simulink model "gnc_ministack"  (R2025a)
settings: Solver=ode45  StartTime=0.0  StopTime=85  RelTol=1e-3
StartFcn:
  | startup()
libraries: sim3dlib x1, aerolibsim3d x1
settings Model: Creator=Jackt  LastModifiedBy=Jackt

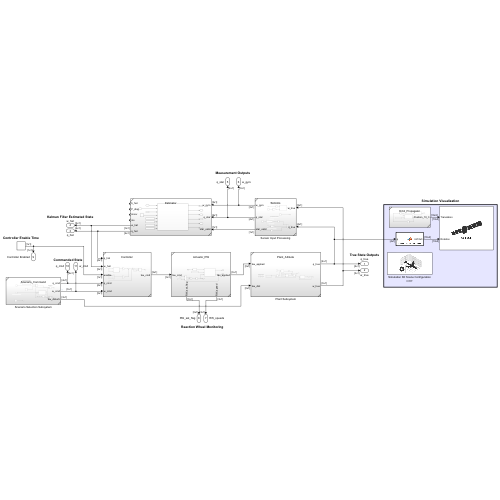
[thumbnail: Simulink's stored preview of the top-level diagram]
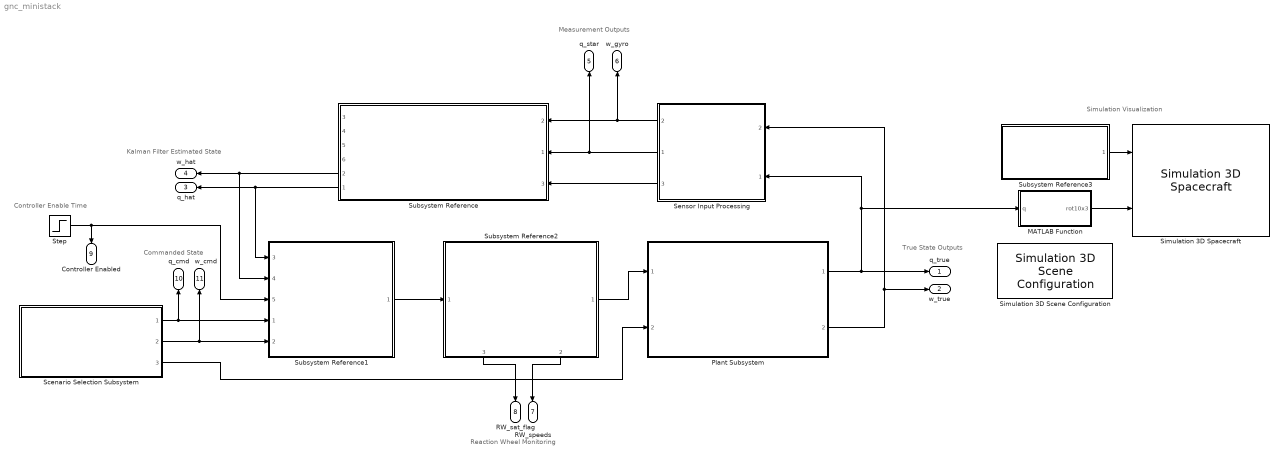
== system gnc_ministack ==
  note: Commanded State
  note: Controller Enable Time
  note: Reaction Wheel Monitoring
  note: Simulation Visualization
  note: Measurement Outputs
  note: True State Outputs
  note: Kalman Filter Estimated State
  MATLAB Function : MATLAB Function  TreatAsAtomicUnit=on
  Plant Subsystem : Subsystem  ReferencedSubsystem=Plant_Attitude
  Scenario Selection Subsystem : Subsystem  ReferencedSubsystem=Scenario_Command
  Sensor Input Processing : Subsystem  ReferencedSubsystem=Sensors
      settings: PortSchema="{\"entries\":[{\"content\":{\"sides\":[{\"content\":{\"connectorIds\":[\"In2\",\"In1\"]},\"type\":\"ConnectorPlacement.EquallySpacedRectSide\",\"uuid\":\"c1e9cccd-a19b-49d9-bc23-c04dc12a4bb5\"},{\"content\":{\"connectorIds\":[\"Out2\",\"Out1\",\"Out3\"],\"side\":\"RIGHT\"},\"type\":\"ConnectorPlacement.EquallySpacedRectSide\",\"uuid\":\"d99cdc6b-e9ef-4ed5-80da-dd2badbe997a\"},{\"content\":{\"side\":\"TOP\"},\"type\":\"ConnectorPlacement.EquallySpacedRectSide\",\"uuid\":\"ee231260-93e9-44f5-bf52-f5add3775a1d\"}]},\"type\":\"ConnectorPlacement.EquallySpacedConnector\",\"uuid\":\"7e127460-3e6f-4f82-b424-e04fed54d7b3\"}],\"packageUris\":[\"http://schema.mathworks.com/mf0/Connector/R2020b\"],\"version\":\"1.0\"}"
  Simulation 3D Scene Configuration : sim3dlib/Simulation 3D Scene Configuration  Priority=0  ProjectFormat=Default Scenes  SceneDesc=Earth  ProjectName=C:\Program Files\MATLAB\R2025a\toolbox\shared\sim3d_projects\automotive_project_windows\UE\WindowsNoEditor\VehicleSimulation.exe  ScenePath=/Game/Maps/HwStrght  EnableOpenDRIVE=off  vehTagList={'Custom';'Scene Origin';'SimulinkVehicle1'}  vehTag=SimulinkVehicle1  AttachedCameraRelativeTranslation=[0 0 0]  FreeCameraDefaultInitialTranslation=[-14000000, 0, 0]  AttachedCameraRelativeRotation=[0 0 0]  FreeCameraDefaultInitialRotation=[0, 0, 0]  ViewpointName=Custom  FreeCameraInitialTranslation=[-6, 0, 2]  ViewpointTranslation=[0 0 0]  FreeCameraInitialRotation=[0, -15, 0]  ViewpointRotation=[0 0 0]  OpVisEn=off  Ts=.02  EnableWindow=on  EnableRemoteAccess=off  EnableWeather=on  SunAzimuth=284.400  SunAltitude=40.0  EnableGeospatialSun=off  Latitude=0  Longitude=0  Date=2023-01-01  Time=10:30:00  GeoTimeZone=-5.0  SunDaylightSaving=off  wind=1  clouds=10  EnableVolumetricClouds=off  CloudCoverage=0  CloudAltitude=6  fog=0  rain=0  RaindropsEffect=off  SnowDensity=0  EnableGeospatial=off  TilesetSource=Earth terrain  UseTrueOrigin=off  OriginHeight=30000  OriginLatitude=40.744652  OriginLongitude=-73.988864  MapStyle=Aerial  AdditionalAssetIDs=[]  UseAdvancedSunSky=off  SolarTime=11  TimeZone=-5  Day=21  Month=9  Year=2022  UseDaylightSavingTime=off  DSTStartDay=10  DSTStartMonth=3  DSTEndDay=3  DSTEndMonth=11  DSTSwitchHour=2  sensorTag=MainCamera1  sensorId=1  sensorName=MainCamera1  mountLoc=Origin  offsetFlag=off  tmountOffset=[0, 0, 0]  rmountOffset=[0, 0, 0]  HorizontalResolution=1280  VerticalResolution=720  HorizontalFOV=60  mountPoint=[0 0 0]  mountOrientation=[0 0 0]  aMode=0  ID=1  GeoTrigger=Inactive  ViewNameList={'Custom'}  ViewTranslationList={'[-6 0 2]'}  ViewRotationList={'[0 -15 0]'}
      settings: AttributesFormatString=ICRF  LibrarySourceBlock=aerolibsim3d/Simulation 3D Scene Configuration
  Simulation 3D Spacecraft : aerolibsim3d/Simulation 3D Spacecraft  Priority=-1  Mesh=CubeSat  MeshPath=/MathWorksAerospaceContent/Vehicles/Spacecraft/CubeSat/Mesh/SK_CubeSat.SK_CubeSat  MeshPathSmall=/MathWorksAerospaceContent/Vehicles/Spacecraft/SmallSat/Mesh/SK_SmallSat.SK_SmallSat  SpacecraftColor=Silver  ActorName=SimulinkVehicle1  Translation=zeros(10, 3)  Rotation=zeros(10, 3)  ScaleInputPort=Dialog  Scale=[1 1 1]  InitialScale=[1 1 1]  IsGHSensorEnabled=off  AreGHRaysVisible=off  IsOutputReshapeEnabled=on  GHRayLength=1524  GHBodyOffset=1  GHContactLocation1=[0 0 0]  GHContactLocation2=[0 0 0]  GHContactLocation3=[0 0 0]  GHContactLocation4=[0 0 0]  WoWSensorTolerance=0.05  SampleTime=-1  ActorType=SimulinkVehicle  ID=1  aMode=0  ActorTag=SimulinkVehicle1
  Step : Step  Time=0  Before=1  SampleTime=0  VectorParams1D=off
  Subsystem Reference : Subsystem  ReferencedSubsystem=Estimator
      settings: PortSchema="{\"entries\":[{\"content\":{\"sides\":[{\"content\":{\"connectorIds\":[\"In2\",\"In1\",\"In3\"]},\"type\":\"ConnectorPlacement.EquallySpacedRectSide\",\"uuid\":\"6ff88212-69d9-4c32-a110-b4128dbcbd58\"},{\"content\":{\"connectorIds\":[\"Out3\",\"Out4\",\"Out5\",\"Out6\",\"Out2\",\"Out1\"],\"side\":\"RIGHT\"},\"type\":\"ConnectorPlacement.EquallySpacedRectSide\",\"uuid\":\"13b22769-b1cf-40a2-97ae-fd353d8761f4\"},{\"content\":{\"side\":\"TOP\"},\"type\":\"ConnectorPlacement.EquallySpacedRectSide\",\"uuid\":\"80c1570c-552a-494f-85a9-3ba650112d27\"}]},\"type\":\"ConnectorPlacement.EquallySpacedConnector\",\"uuid\":\"37c5906b-3676-4ab4-a32b-12b3e3b6617e\"}],\"packageUris\":[\"http://schema.mathworks.com/mf0/Connector/R2020b\"],\"version\":\"1.0\"}"
  Subsystem Reference1 : Subsystem  ReferencedSubsystem=Controller
      settings: PortSchema="{\"entries\":[{\"content\":{\"sides\":[{\"content\":{\"connectorIds\":[\"In3\",\"In4\",\"In5\",\"In1\",\"In2\"]},\"type\":\"ConnectorPlacement.EquallySpacedRectSide\",\"uuid\":\"50b51f02-92a3-4895-831f-474087d70428\"},{\"content\":{\"connectorIds\":[\"Out1\"],\"side\":\"RIGHT\"},\"type\":\"ConnectorPlacement.EquallySpacedRectSide\",\"uuid\":\"95d54d9e-6673-49b8-8b0a-15f9a2d5d6ed\"},{\"content\":{\"side\":\"TOP\"},\"type\":\"ConnectorPlacement.EquallySpacedRectSide\",\"uuid\":\"9b2dfc11-3477-4b71-bffc-31b65fad140d\"}]},\"type\":\"ConnectorPlacement.EquallySpacedConnector\",\"uuid\":\"333a9d20-5e34-4443-bcbe-37e2758feffc\"}],\"packageUris\":[\"http://schema.mathworks.com/mf0/Connector/R2020b\"],\"version\":\"1.0\"}"
  Subsystem Reference2 : Subsystem  ReferencedSubsystem=Actuator_RW
      settings: PortSchema="{\"entries\":[{\"content\":{\"sides\":[{\"content\":{\"connectorIds\":[\"In1\"]},\"type\":\"ConnectorPlacement.EquallySpacedRectSide\",\"uuid\":\"970f40e1-f7ca-420b-8ec9-a2b921625748\"},{\"content\":{\"connectorIds\":[\"Out1\"],\"side\":\"RIGHT\"},\"type\":\"ConnectorPlacement.EquallySpacedRectSide\",\"uuid\":\"35de2d62-f31e-438d-9acc-19246649a370\"},{\"content\":{\"side\":\"TOP\"},\"type\":\"ConnectorPlacement.EquallySpacedRectSide\",\"uuid\":\"82a92509-4f7d-481c-8e84-283404e2f7d8\"},{\"content\":{\"connectorIds\":[\"Out3\",\"Out2\"],\"side\":\"BOTTOM\"},\"type\":\"ConnectorPlacement.EquallySpacedRectSide\",\"uuid\":\"b07604dc-8104-479b-9fb4-03ecbc98cb9a\"}]},\"type\":\"ConnectorPlacement.EquallySpacedConnector\",\"uuid\":\"d401c8d7-6003-4b17-a86f-c889bdabed91\"}],\"packageUris\":[\"http://schema.mathworks.com/mf0/Connector/R2020b\"],\"version\":\"1.0\"}"
  Subsystem Reference3 : Subsystem  ReferencedSubsystem=Orbit_Propagator
  q_true : Outport
  w_true : Outport  Port=2
  q_hat : Outport  Port=3
  w_hat : Outport  Port=4
  q_star : Outport  Port=5
  w_gyro : Outport  Port=6
  RW_speeds : Outport  Port=7
  RW_sat_flag : Outport  Port=8
  Controller Enabled : Outport  Port=9
  q_cmd : Outport  Port=10
  w_cmd : Outport  Port=11
  wires:
  Plant Subsystem/1 -> Sensor Input Processing/1, MATLAB Function/1(q), q_true/1
  Plant Subsystem/2 -> w_true/1, Sensor Input Processing/2
  Scenario Selection Subsystem/1 -> Subsystem Reference1/1, q_cmd/1
  Scenario Selection Subsystem/2 -> w_cmd/1, Subsystem Reference1/2
  Subsystem Reference1/1 -> Subsystem Reference2/1
  Scenario Selection Subsystem/3 -> Plant Subsystem/2
  Sensor Input Processing/1 -> q_star/1, Subsystem Reference/1
  Sensor Input Processing/2 -> Subsystem Reference/2, w_gyro/1
  Sensor Input Processing/3 -> Subsystem Reference/3
  Subsystem Reference/1 -> Subsystem Reference1/3, q_hat/1
  Subsystem Reference/2 -> Subsystem Reference1/4, w_hat/1
  Subsystem Reference2/1 -> Plant Subsystem/1
  Subsystem Reference2/2 -> RW_speeds/1
  Subsystem Reference2/3 -> RW_sat_flag/1
  Step/1 -> Subsystem Reference1/5, Controller Enabled/1
  MATLAB Function/1(rot10x3) -> Simulation 3D Spacecraft/2
  Subsystem Reference3/1 -> Simulation 3D Spacecraft/1

== matlab function gnc_ministack/MATLAB Function ==
  data: q input; rot10x3 output
function rot10x3 = pack_cubesat_rpy(q)
% q: [4x1] scalar-first quaternion (assumed unit-ish)
% rot10x3: [10x3] rows are bones; row1 is BODY [roll pitch yaw] rad

q = q(:);
q = q / max(norm(q), 1e-12);

% Optional: stabilize sign to reduce visual "flips"
if q(1) < 0
    q = -q;
end

% Convert quaternion -> roll/pitch/yaw (ZYX yaw-pitch-roll)
q0=q(1); q1=q(2); q2=q(3); q3=q(4);

% yaw (psi)
psi = atan2(2*(q0*q3 + q1*q2), 1 - 2*(q2^2 + q3^2));
% pitch (theta)
s = 2*(q0*q2 - q3*q1);
s = min(max(s, -1), 1);
theta = asin(s);
% roll (phi)
phi = atan2(2*(q0*q1 + q2*q3), 1 - 2*(q1^2 + q2^2));

rot10x3 = zeros(10,3);
rot10x3(1,:) = [phi, theta, psi];
end
